simulink model "test1"  (R2022b)
settings: Solver=FixedStepDiscrete  StartTime=0.0  StopTime=10  FixedStep=0.002  RelTol=1e-3
undefined symbols (not defined in the file or in its folder): DiscIntNeverNeededParam, Discrete, Time
libraries: ctrlSharedLib x1
settings Model: Creator=19114  LastModifiedBy=19114

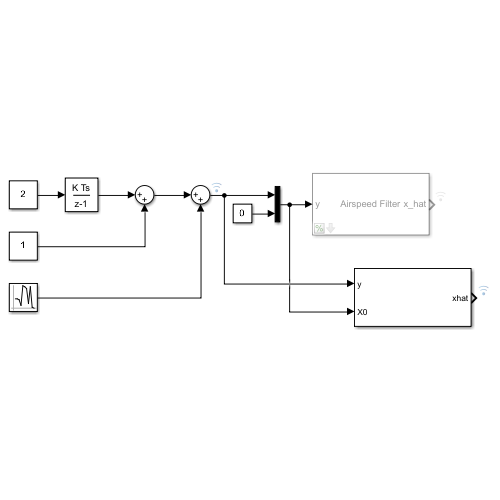
[thumbnail: Simulink's stored preview of the top-level diagram]
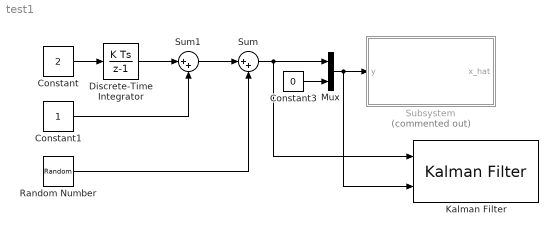
== system test1 ==
  Constant : Constant  Value=2
  Constant1 : Constant
  Constant3 : Constant  Value=0  OutDataTypeStr=double  LockScale=on
  Discrete-Time Integrator : DiscreteIntegrator  SampleTime=-1  ICPrevOutput=DiscIntNeverNeededParam  ICPrevScaledInput=DiscIntNeverNeededParam
  Kalman Filter : ctrlSharedLib/Kalman Filter  TimeDomain=Discrete-Time  UseCurrentEstimator=off  ModelSource=Individual A, B, C, D matrices  ModelSourceVariable=ss(0.95,1,1,0,1)  A=[1 0.002;0 1]  B=1  C=[1 0]  D=0  NumberOfStates=1  NumberOfInputs=1  NumberOfOutputs=1  InitialEstimateSource=Input port  X0=0  P0=10  UseK=off  UseGH=off  NumberOfProcessNoiseInputs=1  G=1  TimeInvariantG=on  H=[1 0]  TimeInvariantH=on  Q=0.2  TimeInvariantQ=on  R=0.2  TimeInvariantR=on  N=0  TimeInvariantN=on  AddInputPort=off  AddEnablePort=off  OutputEstimatedY=off  OutputP=off  Ts=-1
  Mux : Mux  Inputs=2
  Random Number : RandomNumber  Variance=0.005  SampleTime=0.002
  Subsystem : Subsystem  Commented=on  mask{r1=0.2, r2=2, q=0.2, dt=0.002}
      mask prompts: r1 "airspeed measurement standard deviation in [m/s]"; r2 "airspeed rate measurement standard deviation in [m/s²]"; q "standard deviation on the airspeed rate deviation in the model in [m/s²]"; dt "SampleTime"
      mask DialogControl DescGroupVar Prompt: Airspeed Filter
      mask DialogControl DescTextVar Prompt: Filter airspeed and rate using a constant airspeed rate model in a steady state Kalman Filter.
      mask DialogControl ParameterGroupVar Prompt: 参数
      mask Display:
      | port_label('input', 1, 'y');
      | port_label('output', 1, 'x_hat');
      | disp('Airspeed Filter');
  Sum : Sum  Inputs=|++
  Sum1 : Sum  Inputs=|++
  wires:
  Constant3/1 -> Mux/2
  Sum1/1 -> Sum/1
  Discrete-Time Integrator/1 -> Sum1/1
  Constant/1 -> Discrete-Time Integrator/1
  Random Number/1 -> Sum/2
  Constant1/1 -> Sum1/2
  Mux/1 -> Kalman Filter/2, Subsystem/1(y)
  Sum/1 -> Kalman Filter/1, Mux/1

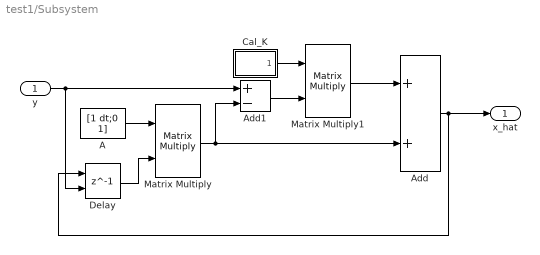
== system test1/Subsystem ==
  y : Inport
  A : Constant  Value=[1 dt;0 1]  OutDataTypeStr=single
  Add : Sum
  Add1 : Sum  Inputs=+-
  "Cal_K " : Subsystem
  Delay : Delay  DelayLength=1  InitialConditionSource=Input port
      settings: InputPortMap=u0,p4
  Matrix Multiply : Product  Multiplication=Matrix(*)
  Matrix Multiply1 : Product  Multiplication=Matrix(*)
  x_hat : Outport
  wires:
  A/1 -> Matrix Multiply/1
  y/1 -> Add1/1, Delay/2
  Matrix Multiply/1 -> Add1/2, Add/2
  Add/1 -> x_hat/1, Delay/1
  "Cal_K "/1(k_gain) -> Matrix Multiply1/1
  Delay/1 -> Matrix Multiply/2
  Add1/1 -> Matrix Multiply1/2
  Matrix Multiply1/1 -> Add/1

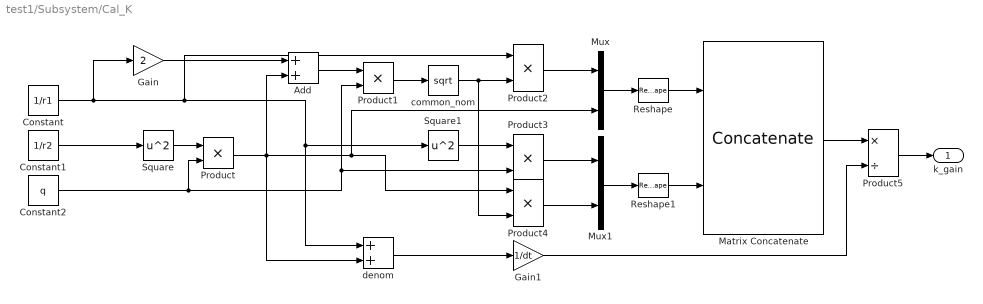
== system test1/Subsystem/Cal_K  ==
  Add : Sum
  Constant : Constant  Value=1/r1  OutDataTypeStr=single
  Constant1 : Constant  Value=1/r2  OutDataTypeStr=single
  Constant2 : Constant  Value=q  OutDataTypeStr=single
  Gain : Gain  Gain=2
  Gain1 : Gain  Gain=1/dt
  Matrix Concatenate : Concatenate  Mode=Multidimensional array
  Mux : Mux  Inputs=2
  Mux1 : Mux  Inputs=2
  Product{,1..4} (5 alike) : Product
  Product5 : Product  Inputs=*/
  Reshape : Reshape  OutputDimensionality=Row vector (2-D)
  Reshape1 : Reshape  OutputDimensionality=Row vector (2-D)
  Square : Math  Operator=square
  Square1 : Math  Operator=square
  common_nom : Sqrt
  denom : Sum
  k_gain : Outport
  wires:
  Constant1/1 -> Square/1
  Square/1 -> Product/1
  Constant2/1 -> Product3/2, Product1/2, Product/2
  Product/1 -> denom/2, Add/2, Product4/1, Mux/2
  Constant/1 -> Gain/1, Product2/1, denom/1, Square1/1
  Gain/1 -> Add/1
  Add/1 -> Product1/1
  Product1/1 -> common_nom/1
  Product2/1 -> Mux/1
  common_nom/1 -> Product4/2, Product2/2
  Mux/1 -> Reshape/1
  Mux1/1 -> Reshape1/1
  Product3/1 -> Mux1/1
  Square1/1 -> Product3/1
  Product4/1 -> Mux1/2
  Matrix Concatenate/1 -> Product5/1
  denom/1 -> Gain1/1
  Product5/1 -> k_gain/1
  Gain1/1 -> Product5/2
  Reshape/1 -> Matrix Concatenate/1
  Reshape1/1 -> Matrix Concatenate/2
